simulink model "House_SFH45"  (Simulink 7.6)
settings: Solver=ode45  StartTime=0.0  StopTime=365*3600*24  RelTol=1e-3
libraries: carnot x20, simulink x3
settings Model: Creator=U_13.adm_zivi  LastModifiedBy=drhf  SimulationMode=accelerator
settings OptimizationCC: ExpressionDepthLimit=128
settings DebuggingCC: FcnCallInpInsideContextMsg=Enable All  StateNameClashWarn=none
settings CodeAppCC: CustomSymbolStrType=$N$R$M_T

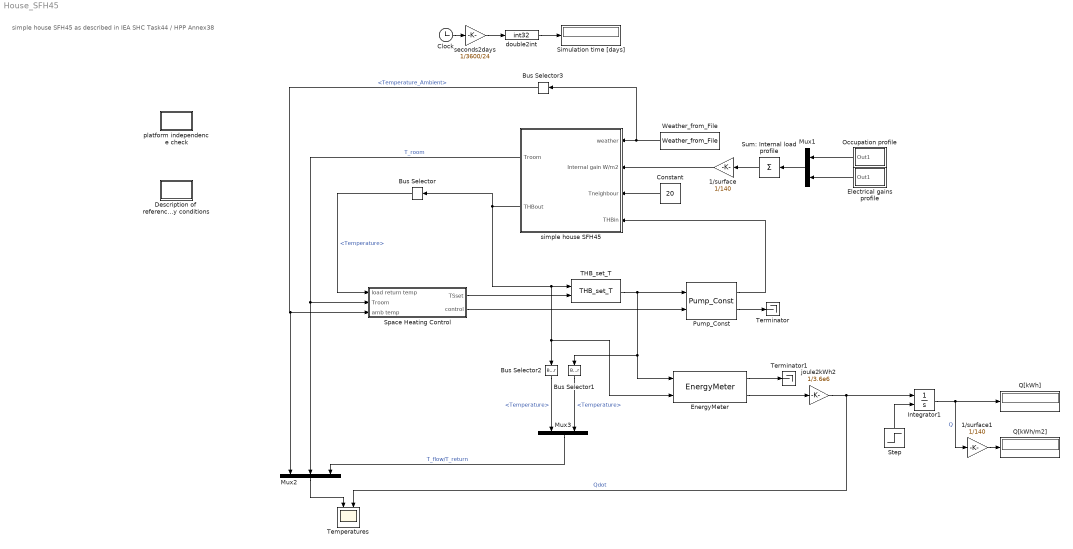
== system House_SFH45 ==
  note: simple house SFH45 as described in IEA SHC Task44 / HPP Annex38
  1/surface : Gain  Gain=1/140
  1/surface1 : Gain  Gain=1/140
  Bus Selector : BusSelector  OutputSignals=Temperature
  Bus Selector1 : BusSelector  OutputSignals=Temperature
  Bus Selector2 : BusSelector  OutputSignals=Temperature
  Bus Selector3 : BusSelector  OutputSignals=Temperature_Ambient
  Clock : Clock
      settings: Decimation=10
  Constant : Constant  Value=20
  "Description of  reference buidling and boundary conditions " : Subsystem
      settings: OpenFcn=|
      | filepath = fullfile(path_carnot('libsl'),'Load','Houses', 'Simple_House_ISO_GroundModel','specification');
      | 
      | open(fullfile(filepath, 'T44A38_Rep_C1_B_ReferenceBuildingDescription_Final_Revised_130906.pdf'));
      | open(fullfile(filepath, 'T44A38_Rep_C1_A_BoundaryConditions_Final_Revised_131108.pdf'));
      mask Display: disp('.pdf')
  Electrical gains profile : Subsystem  mask{period=24*3600, rep_seq_t=[0 1 6 7 8 9 11 12 13 18 19 20 22 23]*3600, rep_seq_d=[1 5 1 1 1 2 1 1 4 2 1 2 1 1]*3600, rep_seq_y=[105 55 392.5 457.5 420 55 250 55 120 170 615 420 442.5 355]}
      mask prompts: period "Timeperiod in s"; rep_seq_t "Time values in s"; rep_seq_d "Duration in s"; rep_seq_y "Output values"
  EnergyMeter : carnot/Control/EnergyMeter  SystemSampleTime=-1
  Integrator1 : Integrator  ExternalReset=rising
  Mux1 : Mux  Inputs=2
  Mux2 : Mux  Inputs=3
  Mux3 : Mux  Inputs=2
  Occupation profile : Subsystem  mask{period=24*3600, rep_seq_t=[0 6 7 8 9 11 12 13 14 15 17 18 20 21 22]*3600, rep_seq_d=[6 1 1 1 2 1 1 1 1 2 1 2 1 1 2]*3600, rep_seq_y=[4 2 3 2 0 1 3 2 1 0 1 2 4 3 4]*60}
      mask prompts: period "Timeperiod in s"; rep_seq_t "Time values in s"; rep_seq_d "Duration in s"; rep_seq_y "Output values"
  Pump_Const : carnot/Hydraulics/Pump_Const  SystemSampleTime=-1  mdotmax=700/3600  dia=0.402  power=81  p0=3e5  fluid_id=Water  mix=0  UA=3  mcp=4000  tamb=20
  Q[kWh/m2] : Display
  Q[kWh] : Display
  Simulation time [days] : Display
  Space Heating Control : Subsystem  mask{Tset=20, Q_LOC=4072, Td_in=35, Td_out=30, Tambd=-10, n_rad=1.1}
      mask prompts: Tset "desired room Temperature [°C]"; Q_LOC "design heat load [W]"; Td_in "design inlet temperature of the heating system [°C]"; Td_out "design outlet temperature of the heating system [°C]"; Tambd "design outdoor temperature"; n_rad "radiatior exponent"
      mask init:
      | dTd = 0.5*(Td_in + Td_out) - Tset;
  Step : Step  Time=0  SampleTime=0
  Sum: Internal load profile : Sum  Inputs=+
  THB_set_T : carnot/Source/Simple/THB_set_T  SystemSampleTime=-1
  Temperatures : Scope  NumInputPorts=2
      settings: TickLabels=on  YMin=-7.5~0  YMax=35~0.0019  Decimation=1000  SampleInput=on  SampleTime=3600*3
  Terminator : Terminator
  Terminator1 : Terminator
  Weather_from_File : carnot/Weather/Weather_from_File  SystemSampleTime=-1  file=FR_Strasbourg  ext=.dat
  double2int : DataTypeConversion  OutDataTypeStr=int32
  joule2kWh2 : Gain  Gain=1/3.6e6
  "platform independence check " : Subsystem
      settings: OpenFcn=open(fullfile(path_carnot('help'), 'pdf', 'Peter_Wintler_Dott_IEA_Task_44_Building_2014.pdf'));
      mask Display: disp('.pdf')
  seconds2days : Gain  Gain=1/3600/24
  simple house SFH45 : Subsystem  mask(simple house){Ahabit=140, Hroom=2.6, UA=[0.197*(54.6+26.4)+0.286*((45.7+56.0)*2 -(12+4+3+4))  70*0.183*0.8  0], Awin=[12 4 3 4], AziWin=[0 90 -180 -90], Uwin=[1    1   1    1]*1.5, Gwin=[1    1   1    1]*0.622*(1-0.15), shade=0.75, tini=20, vent=0.4, rec=0, mc=0.5e6*140 % 0.5 MJ/m2/K, uaheating=425 %400, dpcoeff=[10 100], heatload=4300, delta_t_nom=15, n_rad=1.1, mass_times_cap=40e6}
      mask prompts: Ahabit "ground surface in m²"; Hroom "height of rooms in m"; UA "heat transfer [to_ambient(walls/roof)  to_ground(floor)  to_neighbour] in W/K"; Awin "surface of 4 windows in m² (vector)"; AziWin "orientation of 4 windows (south 0, east -90,west 90)"; Uwin "heat loss coefficient 4 windows in W/m²/K [vector]"; Gwin "light transmittance 4 windows (0..1) * (1 - frame_part) [vector]"; shade "shading factor [0..1] when T room > 4 K + T_init"; tini "initial temperature"; vent "ventilation rate in 1/h"; rec "heat recovery (0..1)"; mc "total thermal capacity in J/K"; uaheating "heat transfer of the heating system in W/K"; dpcoeff "pressure drop coefficients [linear quadratic] in Pa/(kg/s), Pa/(kg/s)²"; heatload "heatload  [W]"; delta_t_nom "nominal temperature difference between desired temperature and incoming THB [K]"; n_rad "radiator exponent"; mass_times_cap "mass*capacity of heating system [J/K]"
      mask help:
      | Simple model of 1-node room or house. The differential equation
      | (m*c)house * dT/dt = solar_gain + internal_gain + heating_power - losses_to_ambient - losses_to_neighbour_room
      | is solved.
      | The heating power is generated by a radiator or floor heating system.
      | The windows have an automatic shading (shading factor) if room temperature rises 4 K above initial temperature.
      | solar gain = Solar_Radiation_on_window * light_transmittance * shading_factor
      | Use "look under mask" to set up the models parameters (initial conditions, surfaces characteristics...).
      | A usual value for the internal gains is 2.3 W/m².
      mask init:
      | invmc = 1/mc;
      | rec = max(0,min(1,rec));
      | Gwin = max(0,min(1,Gwin));
      | shade = max(0, min(1, shade));
      | UAout = UA(1);
      | UAground = UA(2);
      | UAin = UA(3);
      mask Help: eval('man(''simple_house'')')
      mask Display: plot(0,-15,80,100,[30,30,60,60,30],[20,50,50,20,20],[47,47,56,56,47],[40,30,30,40,40],[42,42,34,34],[20,40,40,20],[62,45,28],[48,70,48])
  wires:
  THB_set_T/1 -> EnergyMeter/1, Bus Selector1/1, Pump_Const/1
  Space Heating Control/1(TSset) -> THB_set_T/2
  Space Heating Control/2(control) -> Pump_Const/2
  Weather_from_File/1 -> simple house SFH45/1(weather), Bus Selector3/1
  Pump_Const/1 -> simple house SFH45/4(THBin)
  simple house SFH45/2(THBout) -> Bus Selector/1, EnergyMeter/2, Bus Selector2/1, THB_set_T/1
  Bus Selector/1 -> Space Heating Control/1(load return temp)  "<Temperature>"
  simple house SFH45/1(Troom) -> Mux2/2, Space Heating Control/2(Troom)  "T_room"
  Pump_Const/2 -> Terminator/1
  Constant/1 -> simple house SFH45/3(Tneighbour)
  Mux1/1 -> Sum: Internal load profile/1
  Occupation profile/1(Out1) -> Mux1/1
  Electrical gains profile/1(Out1) -> Mux1/2
  1/surface/1 -> simple house SFH45/2(Internal gain W/m2)
  Sum: Internal load profile/1 -> 1/surface/1
  Bus Selector3/1 -> Space Heating Control/3(amb temp), Mux2/1  "<Temperature_Ambient>"
  Clock/1 -> seconds2days/1
  seconds2days/1 -> double2int/1
  double2int/1 -> Simulation time [days]/1
  Mux2/1 -> Temperatures/1
  Mux3/1 -> Mux2/3  "T_flow/T_return"
  Bus Selector2/1 -> Mux3/1  "<Temperature>"
  Bus Selector1/1 -> Mux3/2  "<Temperature>"
  EnergyMeter/1 -> Terminator1/1
  EnergyMeter/2 -> joule2kWh2/1
  1/surface1/1 -> Q[kWh/m2]/1
  Integrator1/1 -> 1/surface1/1, Q[kWh]/1  "Q"
  joule2kWh2/1 -> Integrator1/1, Temperatures/2  "Qdot"
  Step/1 -> Integrator1/2

== system House_SFH45/Description of  reference buidling and boundary conditions  ==

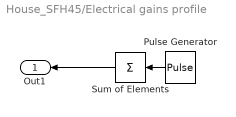
== system House_SFH45/Electrical gains profile ==
  Pulse Generator : DiscretePulseGenerator  PulseType=Time based  Amplitude=rep_seq_y  Period=period  PulseWidth=rep_seq_d*100/period  PhaseDelay=rep_seq_t
  Sum of Elements : Sum  Inputs=+
  Out1 : Outport
  wires:
  Sum of Elements/1 -> Out1/1
  Pulse Generator/1 -> Sum of Elements/1

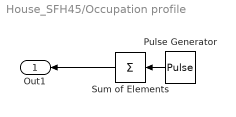
== system House_SFH45/Occupation profile ==
  Pulse Generator : DiscretePulseGenerator  PulseType=Time based  Amplitude=rep_seq_y  Period=period  PulseWidth=rep_seq_d*100/period  PhaseDelay=rep_seq_t
  Sum of Elements : Sum  Inputs=+
  Out1 : Outport
  wires:
  Sum of Elements/1 -> Out1/1
  Pulse Generator/1 -> Sum of Elements/1

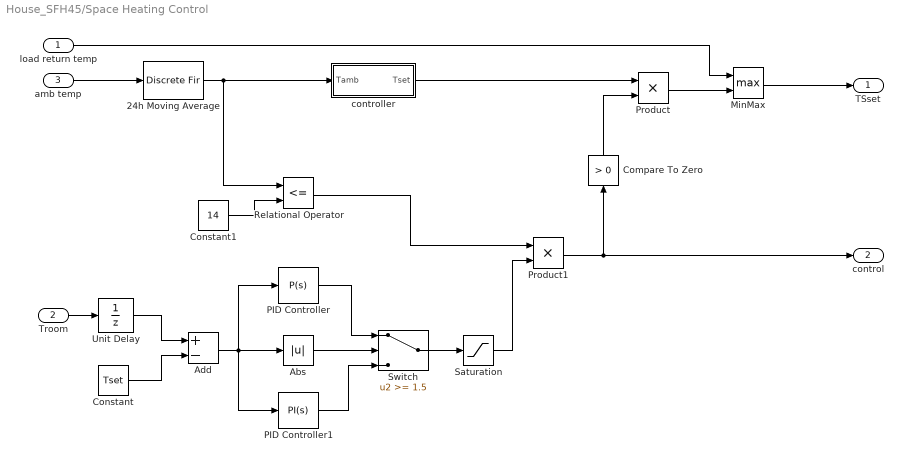
== system House_SFH45/Space Heating Control ==
  load return temp : Inport
  Troom : Inport  Port=2
  amb temp : Inport  Port=3
  24h Moving Average : DiscreteFir  NumCoeffs=ones(1,24)*(1/24)  SampleTime=3600  RndMeth=Nearest
  Abs : Abs
  Add : Sum  Inputs=+-
  Compare To Zero : simulink/Logic and Bit Operations/Compare To Zero  SystemSampleTime=-1  relop=>  LogicOutDataTypeMode=boolean
  Constant : Constant  Value=Tset
  Constant1 : Constant  Value=14
  MinMax : MinMax  Function=max  Inputs=2
  PID Controller : simulink/Continuous/PID Controller  DialogController=pidpack.PIDConfig.pidDDGCreate  DialogControllerArgs=DataTag0  SystemSampleTime=-1  Controller=P  TimeDomain=Continuous-time  SampleTime=1  IntegratorMethod=Forward Euler  FilterMethod=Forward Euler  Form=Parallel  P=-0.5  I=1  D=0  N=100  InitialConditionSource=internal  InitialConditionForIntegrator=0  InitialConditionForFilter=0  ExternalReset=none  ZeroCross=off  LimitOutput=on  UpperSaturationLimit=1  LowerSaturationLimit=0  LinearizeAsGain=off  AntiWindupMode=none  Kb=1  TrackingMode=off  Kt=1  PParamMin=[]  PParamMax=[]  IParamMin=[]  IParamMax=[]  DParamMin=[]  DParamMax=[]  NParamMin=[]  NParamMax=[]  KbParamMin=[]  KbParamMax=[]  KtParamMin=[]  KtParamMax=[]  POutMin=[]  POutMax=[]  IOutMin=[]  IOutMax=[]  DOutMin=[]  DOutMax=[]  NOutMin=[]  NOutMax=[]  KbOutMin=[]  KbOutMax=[]  KtOutMin=[]  KtOutMax=[]  IntegratorOutMin=[]  IntegratorOutMax=[]  FilterOutMin=[]  FilterOutMax=[]  SumOutMin=[]  SumOutMax=[]  SumI1OutMin=[]  SumI1OutMax=[]  SumI2OutMin=[]  SumI2OutMax=[]  SumI3OutMin=[]  SumI3OutMax=[]  SumDOutMin=[]  SumDOutMax=[]  SaturationOutMin=[]  SaturationOutMax=[]  IntegratorContinuousStateAttributes=''  IntegratorStateMustResolveToSignalObject=off  IntegratorRTWStateStorageClass=Auto  FilterContinuousStateAttributes=''  FilterStateMustResolveToSignalObject=off  FilterRTWStateStorageClass=Auto
  PID Controller1 : simulink/Continuous/PID Controller  DialogController=pidpack.PIDConfig.pidDDGCreate  DialogControllerArgs=DataTag1  SystemSampleTime=-1  Controller=PI  TimeDomain=Continuous-time  SampleTime=1  IntegratorMethod=Forward Euler  FilterMethod=Forward Euler  Form=Parallel  P=-0.8  I=-0.05/3600  D=0  N=100  InitialConditionSource=internal  InitialConditionForIntegrator=0  InitialConditionForFilter=0  ExternalReset=none  ZeroCross=off  LimitOutput=on  UpperSaturationLimit=1  LowerSaturationLimit=0  LinearizeAsGain=off  AntiWindupMode=back-calculation  Kb=1  TrackingMode=off  Kt=1  PParamMin=[]  PParamMax=[]  IParamMin=[]  IParamMax=[]  DParamMin=[]  DParamMax=[]  NParamMin=[]  NParamMax=[]  KbParamMin=[]  KbParamMax=[]  KtParamMin=[]  KtParamMax=[]  POutMin=[]  POutMax=[]  IOutMin=[]  IOutMax=[]  DOutMin=[]  DOutMax=[]  NOutMin=[]  NOutMax=[]  KbOutMin=[]  KbOutMax=[]  KtOutMin=[]  KtOutMax=[]  IntegratorOutMin=[]  IntegratorOutMax=[]  FilterOutMin=[]  FilterOutMax=[]  SumOutMin=[]  SumOutMax=[]  SumI1OutMin=[]  SumI1OutMax=[]  SumI2OutMin=[]  SumI2OutMax=[]  SumI3OutMin=[]  SumI3OutMax=[]  SumDOutMin=[]  SumDOutMax=[]  SaturationOutMin=[]  SaturationOutMax=[]  IntegratorContinuousStateAttributes=''  IntegratorStateMustResolveToSignalObject=off  IntegratorRTWStateStorageClass=Auto  FilterContinuousStateAttributes=''  FilterStateMustResolveToSignalObject=off  FilterRTWStateStorageClass=Auto
  Product : Product
  Product1 : Product
  Relational Operator : RelationalOperator  Operator=<=  OutDataTypeStr=boolean
  Saturation : Saturate  UpperLimit=1  LowerLimit=0  ZeroCross=off
  Switch : Switch  Threshold=1.5
  Unit Delay : UnitDelay  SampleTime=60
  controller : Subsystem
  TSset : Outport
  control : Outport  Port=2
  wires:
  amb temp/1 -> 24h Moving Average/1
  MinMax/1 -> TSset/1
  Troom/1 -> Unit Delay/1
  Constant1/1 -> Relational Operator/2
  Unit Delay/1 -> Add/1
  Constant/1 -> Add/2
  Add/1 -> PID Controller/1, PID Controller1/1, Abs/1
  Abs/1 -> Switch/2
  PID Controller/1 -> Switch/1
  PID Controller1/1 -> Switch/3
  Switch/1 -> Saturation/1
  Saturation/1 -> Product1/2
  Relational Operator/1 -> Product1/1
  Product/1 -> MinMax/2
  load return temp/1 -> MinMax/1
  Product1/1 -> control/1, Compare To Zero/1
  Compare To Zero/1 -> Product/2
  24h Moving Average/1 -> Relational Operator/1, controller/1(Tamb)
  controller/1(Tset) -> Product/1

== system House_SFH45/platform independence check  ==

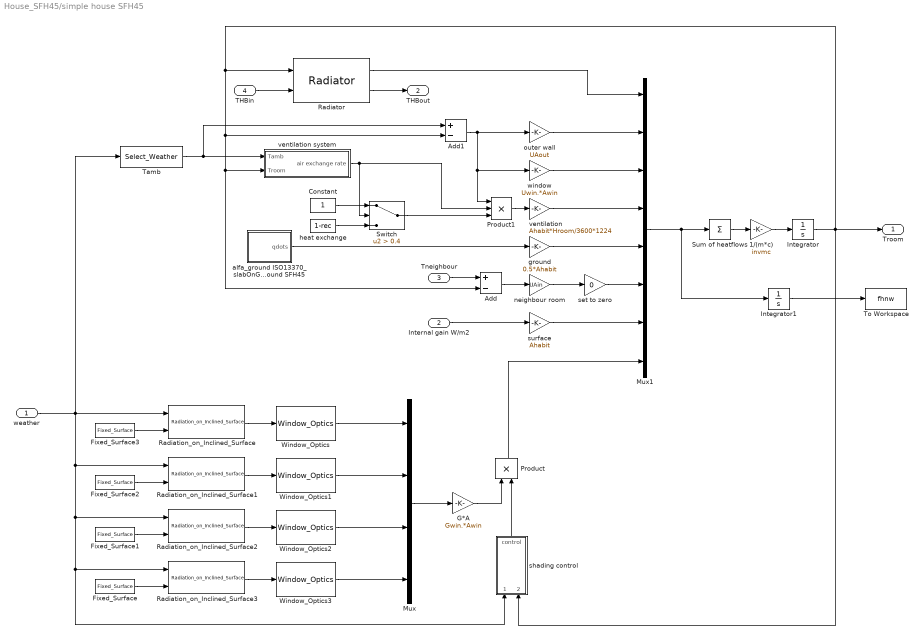
== system House_SFH45/simple house SFH45 ==
  weather : Inport
  Internal gain W/m2 : Inport  Port=2
  Tneighbour : Inport  Port=3
  THBin : Inport  Port=4
  1/(m*c) : Gain  Gain=invmc
  Add : Sum  Inputs=+-
  Add1 : Sum  Inputs=+-
  Constant : Constant
  Fixed_Surface : carnot/Weather/Fixed_Surface  SystemSampleTime=-1  colangle=90  colazi=AziWin(4)  colrot=0
  Fixed_Surface1 : carnot/Weather/Fixed_Surface  SystemSampleTime=-1  colangle=90  colazi=AziWin(3)  colrot=0
  Fixed_Surface2 : carnot/Weather/Fixed_Surface  SystemSampleTime=-1  colangle=90  colazi=AziWin(2)  colrot=0
  Fixed_Surface3 : carnot/Weather/Fixed_Surface  SystemSampleTime=-1  colangle=90  colazi=AziWin(1)  colrot=0
  G*A : Gain  Gain=Gwin.*Awin
  Integrator : Integrator  InitialCondition=tini
  Integrator1 : Integrator
  Mux : Mux
  Mux1 : Mux  Inputs=8
  Product : Product
  Product1 : Product  Inputs=3
  Radiation_on_Inclined_Surface{,1..3} (4 alike) : carnot/Weather/Radiation_on_Inclined_Surface  SystemSampleTime=-1  sky=Perez 1990  reflect=0.2
  Radiator : carnot/Source/Heat_Exchanger/Radiator  SystemSampleTime=-1  pnom=heatload*1.3  dtnom=delta_t_nom  expo=n_rad  mcap=mass_times_cap  tini=tini  lin=0  qua=1000
  Sum of heatflows : Sum  Inputs=+
  Switch : Switch  Criteria=u2 > Threshold  Threshold=0.4
  Tamb : carnot/Weather/Select_Weather  SystemSampleTime=-1  v=6
  To Workspace : ToWorkspace  VariableName=fhnw  SampleTime=3600  SaveFormat=Array
  Window_Optics{,1..3} (4 alike) : carnot/Load/Houses/wall_floor/Window_Optics  SystemSampleTime=-1
  alfa_ground ISO13370_slabOnGround SFH45 : Subsystem  mask(ALFA){wallsize=[7 10], gammat=0, Tmeaninside=23.8, deltathetai=3.8, Tmeanoutside=11, deltathetae=9.3, tshift=319*3600, dwall=0.4, cond_ground=2.0, cp_ground=800, rho_ground=2500, rtot=1./0.183}
      mask prompts: wallsize "size of slab [m] [length width]"; gammat "linear thermal transmittance associated with wall/floor junctions [W/mK]"; Tmeaninside "mean inside temperature over one year [°C]"; deltathetai "amplitude of monthly mean internal temperature [°C]"; Tmeanoutside "mean outside temperature over one year [°C]"; deltathetae "amplitude of monthly mean outside temperature [°C]"; tshift "time shift where external temperature sine-curve shows a mimimum [h]"; dwall "average thickness of side walls inlcuding all layers [m]"; cond_ground "conductivity of ground [W/(m*K)]"; cp_ground "capacity of ground [J/(kg*K)]"; rho_ground "density of ground [kg/m^3]"; rtot "total thermal resistance between driving temperature and ground [mK/W]"
      mask help:
      | Ground heat transfer for a floor "SLAB ON GROUND" according to ISO 13370:2007.
      |
      | qdots : specific heat flow into wall construction, W/m^2,
  ground : Gain  Gain=0.5*Ahabit
  heat exchange : Constant  Value=1-rec
  neighbour room : Gain  Gain=UAin
  outer wall : Gain  Gain=UAout
  set to zero : Gain  Gain=0
  shading control : Subsystem
  surface : Gain  Gain=Ahabit
  ventilation : Gain  Gain=Ahabit*Hroom/3600*1224
  ventilation system : Subsystem
  window : Gain  Gain=Uwin.*Awin
  Troom : Outport
  THBout : Outport  Port=2
  wires:
  Fixed_Surface1/1 -> Radiation_on_Inclined_Surface2/2
  Fixed_Surface3/1 -> Radiation_on_Inclined_Surface/2
  Fixed_Surface/1 -> Radiation_on_Inclined_Surface3/2
  Radiation_on_Inclined_Surface1/1 -> Window_Optics1/1
  Fixed_Surface2/1 -> Radiation_on_Inclined_Surface1/2
  Radiation_on_Inclined_Surface3/1 -> Window_Optics3/1
  weather/1 -> shading control/1(weather), Radiation_on_Inclined_Surface3/1, Radiation_on_Inclined_Surface2/1, Radiation_on_Inclined_Surface1/1, Tamb/1, Radiation_on_Inclined_Surface/1
  Radiation_on_Inclined_Surface2/1 -> Window_Optics2/1
  Window_Optics/1 -> Mux/1
  Window_Optics3/1 -> Mux/4
  Window_Optics1/1 -> Mux/2
  Window_Optics2/1 -> Mux/3
  Mux/1 -> G*A/1
  G*A/1 -> Product/1
  shading control/1(control) -> Product/2
  Internal gain W/m2/1 -> surface/1
  surface/1 -> Mux1/7
  Sum of heatflows/1 -> 1/(m*c)/1
  1/(m*c)/1 -> Integrator/1
  Add/1 -> neighbour room/1
  Product1/1 -> ventilation/1
  Add1/1 -> Product1/1, window/1, outer wall/1
  Tamb/1 -> ventilation system/1(Tamb), Add1/1
  ventilation system/1(air exchange rate) -> Switch/2, Product1/2
  Switch/1 -> Product1/3
  heat exchange/1 -> Switch/3
  Constant/1 -> Switch/1
  alfa_ground ISO13370_slabOnGround SFH45/1(qdots) -> ground/1
  THBin/1 -> Radiator/2
  Radiator/2 -> THBout/1
  Radiator/1 -> Mux1/1
  outer wall/1 -> Mux1/2
  ground/1 -> Mux1/5
  set to zero/1 -> Mux1/6
  Product/1 -> Mux1/8
  neighbour room/1 -> set to zero/1
  Mux1/1 -> Sum of heatflows/1, Integrator1/1
  window/1 -> Mux1/3
  ventilation/1 -> Mux1/4
  Radiation_on_Inclined_Surface/1 -> Window_Optics/1
  Tneighbour/1 -> Add/1
  Integrator/1 -> Radiator/1, Add1/2, Add/2, ventilation system/2(Troom), Troom/1, shading control/2(Troom)
  Integrator1/1 -> To Workspace/1

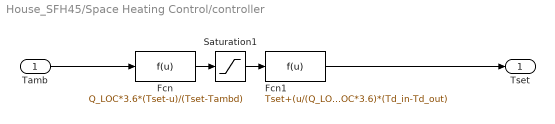
== system House_SFH45/Space Heating Control/controller ==
  Tamb : Inport
  Fcn : Fcn  Expr=Q_LOC*3.6*(Tset-u)/(Tset-Tambd)
  Fcn1 : Fcn  Expr=Tset+(u/(Q_LOC*3.6))^(1/n_rad)*dTd+u/(2*Q_LOC*3.6)*(Td_in-Td_out)
  Saturation1 : Saturate  UpperLimit=inf  LowerLimit=0
  Tset : Outport
  wires:
  Tamb/1 -> Fcn/1
  Fcn/1 -> Saturation1/1
  Fcn1/1 -> Tset/1
  Saturation1/1 -> Fcn1/1

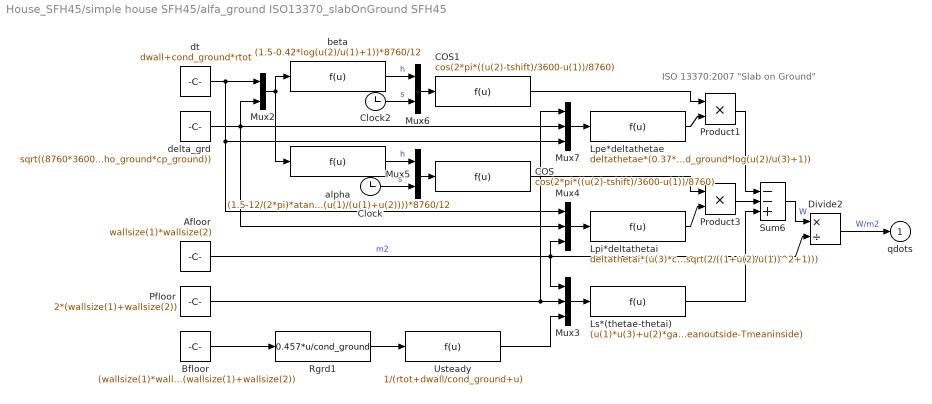
== system House_SFH45/simple house SFH45/alfa_ground ISO13370_slabOnGround SFH45 ==
  note: ISO 13370:2007 "Slab on Ground"
  Afloor : Constant  Value=wallsize(1)*wallsize(2)
  Bfloor : Constant  Value=(wallsize(1)*wallsize(2))/(wallsize(1)+wallsize(2))
  COS : Fcn  Expr=cos(2*pi*((u(2)-tshift)/3600-u(1))/8760)
  COS1 : Fcn  Expr=cos(2*pi*((u(2)-tshift)/3600-u(1))/8760)
  Clock : Clock
      settings: Decimation=10
  Clock2 : Clock
      settings: Decimation=10
  Divide2 : Product  Inputs=*/
  Lpe*deltathetae : Fcn  Expr=deltathetae*(0.37*u(1)*cond_ground*log(u(2)/u(3)+1))
  Lpi*deltathetai : Fcn  Expr=deltathetai*(u(3)*cond_ground/u(1)*sqrt(2/((1+u(2)/u(1))^2+1)))
  Ls*(thetae-thetai) : Fcn  Expr=(u(1)*u(3)+u(2)*gammat)*(Tmeanoutside-Tmeaninside)
  Mux2 : Mux  Inputs=2
  Mux3 : Mux  Inputs=3
  Mux4 : Mux  Inputs=3
  Mux5 : Mux  Inputs=2
  Mux6 : Mux  Inputs=2
  Mux7 : Mux  Inputs=3
  Pfloor : Constant  Value=2*(wallsize(1)+wallsize(2))
  Product1 : Product  SaturateOnIntegerOverflow=on  RndMeth=Zero  InputSameDT=on  OutDataTypeStr=Inherit: Same as first input
  Product3 : Product  SaturateOnIntegerOverflow=on  RndMeth=Zero  InputSameDT=on  OutDataTypeStr=Inherit: Same as first input
  Rgrd1 : Fcn  Expr=0.457*u/cond_ground
  Sum6 : Sum  Inputs=--+
  Usteady : Fcn  Expr=1/(rtot+dwall/cond_ground+u)
  alpha : Fcn  Expr=(1.5-12/(2*pi)*atan(u(1)/(u(1)+u(2))))*8760/12
  beta : Fcn  Expr=(1.5-0.42*log(u(2)/u(1)+1))*8760/12
  delta_grd : Constant  Value=sqrt((8760*3600*cond_ground)/(pi*rho_ground*cp_ground))
  dt : Constant  Value=dwall+cond_ground*rtot
  qdots : Outport  InitialOutput=0
  wires:
  Divide2/1 -> qdots/1  "W/m2"
  Rgrd1/1 -> Usteady/1
  Bfloor/1 -> Rgrd1/1
  dt/1 -> Mux2/1, Mux4/1, Mux7/3
  delta_grd/1 -> Mux4/2, Mux7/2, Mux2/2
  Mux2/1 -> alpha/1, beta/1
  Mux3/1 -> Ls*(thetae-thetai)/1
  Afloor/1 -> Mux4/3, Divide2/2, Mux3/1  "m2"
  Pfloor/1 -> Mux3/2, Mux7/1
  Usteady/1 -> Mux3/3
  Mux4/1 -> Lpi*deltathetai/1
  Lpi*deltathetai/1 -> Product3/2
  alpha/1 -> Mux5/1  "h"
  Clock/1 -> Mux5/2  "s"
  Mux5/1 -> COS/1
  COS/1 -> Product3/1
  Product3/1 -> Sum6/2
  Ls*(thetae-thetai)/1 -> Sum6/3
  beta/1 -> Mux6/1  "h"
  Clock2/1 -> Mux6/2  "s"
  Mux6/1 -> COS1/1
  COS1/1 -> Product1/1
  Lpe*deltathetae/1 -> Product1/2
  Product1/1 -> Sum6/1
  Mux7/1 -> Lpe*deltathetae/1
  Sum6/1 -> Divide2/1  "W"

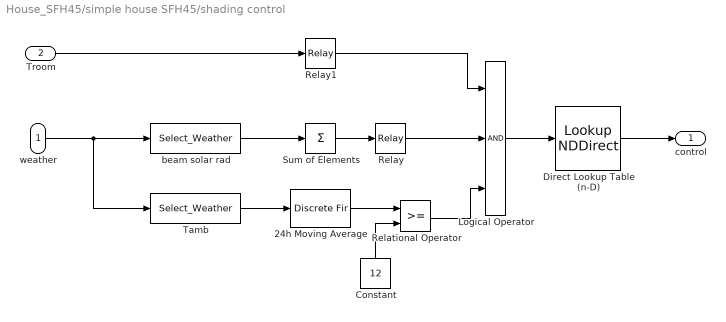
== system House_SFH45/simple house SFH45/shading control ==
  weather : Inport
  Troom : Inport  Port=2
  24h Moving Average : DiscreteFir  NumCoeffs=ones(1,24)*(1/24)  SampleTime=60  RndMeth=Nearest
  Constant : Constant  Value=12
  Direct Lookup Table (n-D) : LookupNDDirect  NumberOfTableDimensions=1  Table=[1 1-shade]
  Logical Operator : Logic  Inputs=3  AllPortsSameDT=off  OutDataTypeStr=boolean
  Relational Operator : RelationalOperator  OutDataTypeStr=boolean
  Relay : Relay  OnSwitchValue=300  OffSwitchValue=200
  Relay1 : Relay  OnSwitchValue=23.8  OffSwitchValue=22.8
  Sum of Elements : Sum  Inputs=+
  Tamb : carnot/Weather/Select_Weather  SystemSampleTime=-1  v=6
  beam solar rad : carnot/Weather/Select_Weather  SystemSampleTime=-1  v=[17 18]
  control : Outport
  wires:
  beam solar rad/1 -> Sum of Elements/1
  24h Moving Average/1 -> Relational Operator/1
  Logical Operator/1 -> Direct Lookup Table (n-D)/1
  Sum of Elements/1 -> Relay/1
  Relay/1 -> Logical Operator/2
  Relational Operator/1 -> Logical Operator/3
  Troom/1 -> Relay1/1
  Direct Lookup Table (n-D)/1 -> control/1
  weather/1 -> Tamb/1, beam solar rad/1
  Relay1/1 -> Logical Operator/1
  Constant/1 -> Relational Operator/2
  Tamb/1 -> 24h Moving Average/1

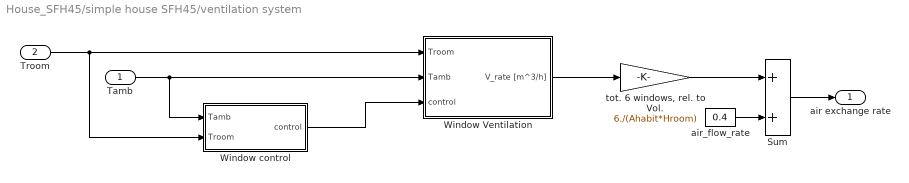
== system House_SFH45/simple house SFH45/ventilation system ==
  Tamb : Inport
  Troom : Inport  Port=2
  Sum : Sum
  Window Ventilation : Subsystem  mask(window ventilation){alpha=10, H=1, W=1}
      mask prompts: alpha "maximal opening angle (°)"; H "height of window (m)"; W "width of window (m)"
      mask help: Simulates the free driven ventilation through a window with an opening angle of [0,1]* max. angle. Valid for angles between 8° and 180°. Output is the VOLUME FLOW RATE in m^3/h. Calculation based on the Ansatz from Weber.
      mask Display: plot(0,10,90,80,[20 70 70 20 20],[20 20 70 70 20],[20 70 80 30 20],[20 20 65 65 20])
  Window control : Subsystem
  air_flow_rate : Constant  Value=0.4
  "tot. 6 windows, rel. to Vol." : Gain  Gain=6./(Ahabit*Hroom)
  air exchange rate : Outport
  wires:
  Window control/1(control) -> Window Ventilation/3(control)
  Window Ventilation/1(V_rate [m^3/h]) -> "tot. 6 windows, rel. to Vol."/1
  air_flow_rate/1 -> Sum/2
  Sum/1 -> air exchange rate/1
  "tot. 6 windows, rel. to Vol."/1 -> Sum/1
  Troom/1 -> Window Ventilation/1(Troom), Window control/2(Troom)
  Tamb/1 -> Window control/1(Tamb), Window Ventilation/2(Tamb)

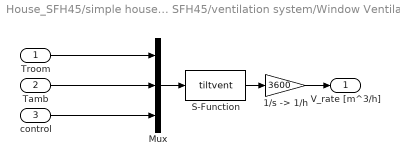
== system House_SFH45/simple house SFH45/ventilation system/Window Ventilation ==
  Troom : Inport
  Tamb : Inport  Port=2
  control : Inport  Port=3
  "1/s -> 1/h" : Gain  Gain=3600
  Mux : Mux  Inputs=3
  S-Function : S-Function  FunctionName=tiltvent  Parameters=alpha, H, W  EnableBusSupport=off
  V_rate [m^3/h] : Outport
  wires:
  Tamb/1 -> Mux/2
  control/1 -> Mux/3
  S-Function/1 -> "1/s -> 1/h"/1
  Mux/1 -> S-Function/1
  Troom/1 -> Mux/1
  "1/s -> 1/h"/1 -> V_rate [m^3/h]/1

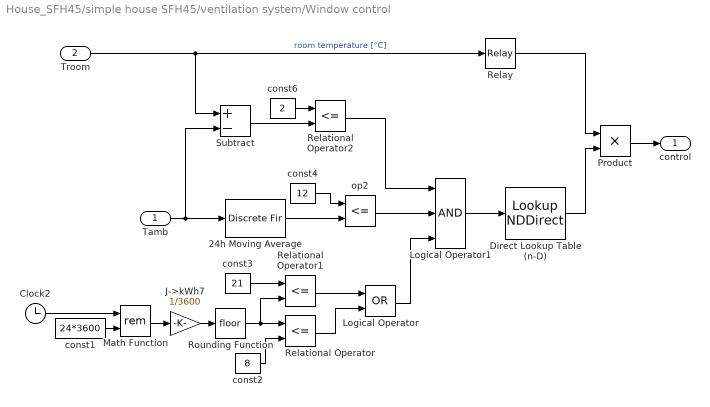
== system House_SFH45/simple house SFH45/ventilation system/Window control ==
  Tamb : Inport
  Troom : Inport  Port=2
  24h Moving Average : DiscreteFir  NumCoeffs=ones(1,24)*(1/24)  SampleTime=3600  RndMeth=Nearest
  Clock2 : Clock
      settings: Decimation=10
  Direct Lookup Table (n-D) : LookupNDDirect  NumberOfTableDimensions=1  Table=[0 1]
  J->kWh7 : Gain  Gain=1/3600  SaturateOnIntegerOverflow=on  OutDataTypeStr=Inherit: Same as input  ParamDataTypeStr=Inherit: Same as input
  Logical Operator : Logic  Operator=OR  AllPortsSameDT=off  OutDataTypeStr=boolean
  Logical Operator1 : Logic  Inputs=3  AllPortsSameDT=off  OutDataTypeStr=boolean
  Math Function : Math  Operator=rem  SaturateOnIntegerOverflow=on
  Product : Product  RndMeth=Zero
  Relational Operator : RelationalOperator  Operator=<=  OutDataTypeStr=boolean
  Relational Operator1 : RelationalOperator  Operator=<=  OutDataTypeStr=boolean
  Relational Operator2 : RelationalOperator  Operator=<=  OutDataTypeStr=boolean
  Relay : Relay  OnSwitchValue=24  OffSwitchValue=23
  Rounding Function : Rounding
  Subtract : Sum  Inputs=+-
  const1 : Constant  Value=24*3600
  const2 : Constant  Value=8
  const3 : Constant  Value=21
  const4 : Constant  Value=12
  const6 : Constant  Value=2
  op2 : RelationalOperator  Operator=<=  OutDataTypeStr=boolean
  control : Outport
  wires:
  Clock2/1 -> Math Function/1
  const1/1 -> Math Function/2
  Math Function/1 -> J->kWh7/1
  J->kWh7/1 -> Rounding Function/1
  Rounding Function/1 -> Relational Operator/1, Relational Operator1/2
  const2/1 -> Relational Operator/2
  const3/1 -> Relational Operator1/1
  Relational Operator1/1 -> Logical Operator/1
  Relational Operator/1 -> Logical Operator/2
  Tamb/1 -> Subtract/2, 24h Moving Average/1
  const4/1 -> op2/1
  Logical Operator/1 -> Logical Operator1/3
  Troom/1 -> Relay/1, Subtract/1  "room temperature [°C]"
  const6/1 -> Relational Operator2/1
  Subtract/1 -> Relational Operator2/2
  Relational Operator2/1 -> Logical Operator1/1
  Logical Operator1/1 -> Direct Lookup Table (n-D)/1
  op2/1 -> Logical Operator1/2
  Direct Lookup Table (n-D)/1 -> Product/2
  Product/1 -> control/1
  Relay/1 -> Product/1
  24h Moving Average/1 -> op2/2
